simulink model "V40AeroDynamics"  (R2017b)
settings: Solver=VariableStepAuto  StartTime=0.0  StopTime=5  RelTol=1e-3
values from neighbouring files (symbols this model uses):
  g = 9.79    [trim_v40.m]
  mass0 = 45    [trim_v40.m]
  p0 = 0    [trim_v40.m]
  pitch0 = 0.0/180*pi    (= 0)    [trim_v40.m]
  q0 = 0    [trim_v40.m]
  r0 = 0    [trim_v40.m]
  rho = 1.213    [trim_v40.m]
  roll0 = 0    [trim_v40.m]
  u0 = Vair0*cos(beta0)*cos(alpha0)    [trim_v40.m]
  v0 = Vair0*sin(beta0)    [trim_v40.m]
  w0 = Vair0*cos(beta0)*sin(alpha0)    [trim_v40.m]
  x0 = 0    [trim_v40.m]
  x_CG = 1.38-0.043    (= 1.337)    [trim_v40.m]
  y0 = 0    [trim_v40.m]
  yaw0 = 0    [trim_v40.m]
  z0 = -200    [trim_v40.m]
  z_CG = 0    [trim_v40.m]
undefined symbols (not defined in the file or in its folder): b_ref, c_bar, CG_ref_x, CG_ref_z, CL0, Clp, Clr, Cm0, Cmq, Cnp, Cnr, CX_d_ca_l, CX_d_ca_r, CX_d_ea_l, CX_d_ea_r, CX_d_r, D_CL_alpha, D_Cm_alpha, DCD_alpha, DCX_beta, Newton, Raphson, S_ref
libraries: simulink_extras x3, shared6dof x1, aerolibasang x1, aerolibtransform2 x1
(part 2 of 2)

== system V40AeroDynamics/Forces & Moments/summation/coef computation4 ==
  In : Inport
  Add1 : Sum  Inputs=++++++++++
  Demux : Demux  Outputs=10
  Out : Outport
  wires:
  Add1/1 -> Out/1
  In/1 -> Demux/1
  Demux/1 -> Add1/1
  Demux/2 -> Add1/2
  Demux/3 -> Add1/3
  Demux/4 -> Add1/4
  Demux/5 -> Add1/5
  Demux/6 -> Add1/6
  Demux/7 -> Add1/7
  Demux/8 -> Add1/8
  Demux/9 -> Add1/9
  Demux/10 -> Add1/10

== system V40AeroDynamics/Forces & Moments/summation/coef computation5 ==
  In : Inport
  Add1 : Sum  Inputs=++++++++
  Demux : Demux  Outputs=8
  Out : Outport
  wires:
  Add1/1 -> Out/1
  In/1 -> Demux/1
  Demux/1 -> Add1/1
  Demux/2 -> Add1/2
  Demux/3 -> Add1/3
  Demux/4 -> Add1/4
  Demux/5 -> Add1/5
  Demux/6 -> Add1/6
  Demux/7 -> Add1/7
  Demux/8 -> Add1/8
